simulink model "Motor_Position"  (R2020a)
settings: Solver=ode15s  StartTime=0.0  StopTime=0.2  RelTol=1e-3
undefined symbols (not defined in the file): b, J, K, Kd, Ki, Kp, L, R, Ts
settings Model: DataDictionary=Motordata.sldd  Creator=NIKITA  LastModifiedBy=NIKITA

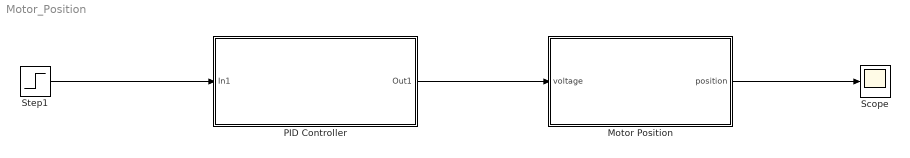
== system Motor_Position ==
  Motor Position : Subsystem
  PID Controller : Subsystem
  Scope : Scope
  Step1 : Step  Time=0  SampleTime=0
  wires:
  Motor Position/1(position) -> Scope/1
  Step1/1 -> PID Controller/1(In1)
  PID Controller/1(Out1) -> Motor Position/1(voltage)

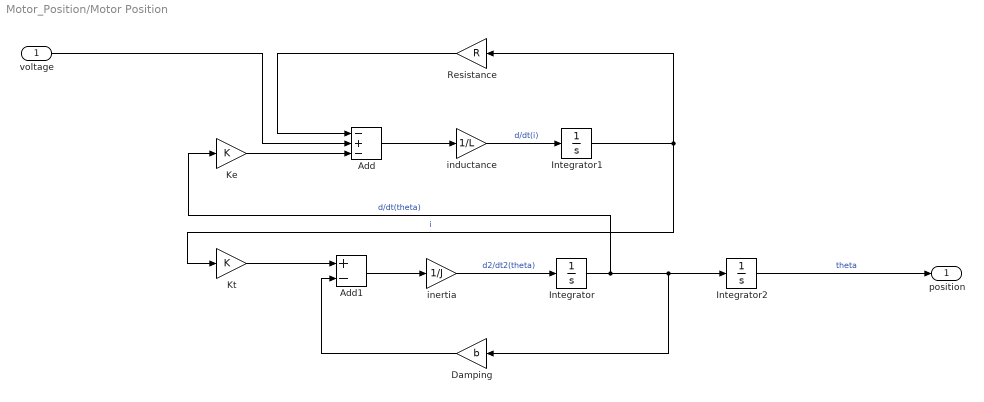
== system Motor_Position/Motor Position ==
  voltage : Inport
  Add : Sum  Inputs=-+-
  Add1 : Sum  Inputs=+-
  Damping : Gain  Gain=b
  "Integrator " : Integrator
  "Integrator1 " : Integrator
  "Integrator2 " : Integrator
  Ke : Gain  Gain=K
  Kt : Gain  Gain=K
  Resistance : Gain  Gain=R
  inductance : Gain  Gain=1/L
  inertia : Gain  Gain=1/J
  position : Outport
  wires:
  Add/1 -> inductance/1
  inertia/1 -> "Integrator "/1  "d2/dt2(theta)"
  Ke/1 -> Add/3
  Damping/1 -> Add1/2
  Resistance/1 -> Add/1
  "Integrator1 "/1 -> Resistance/1, Kt/1  "i"
  Kt/1 -> Add1/1
  "Integrator "/1 -> Ke/1, "Integrator2 "/1, Damping/1  "d/dt(theta)"
  voltage/1 -> Add/2
  inductance/1 -> "Integrator1 "/1  "d/dt(i)"
  Add1/1 -> inertia/1
  "Integrator2 "/1 -> position/1  "theta"

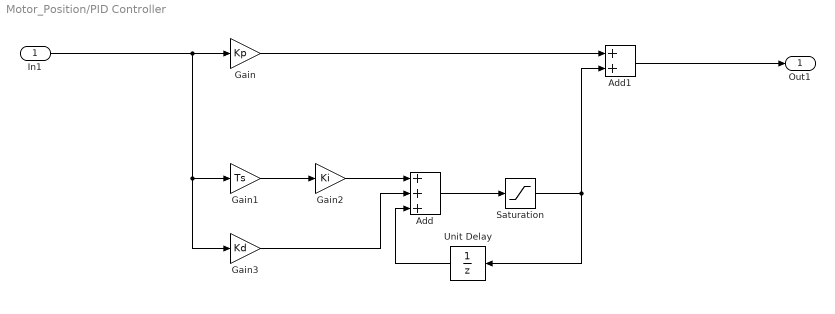
== system Motor_Position/PID Controller ==
  In1 : Inport
  Add : Sum  Inputs=+++
  Add1 : Sum
  Gain : Gain  Gain=Kp
  Gain1 : Gain  Gain=Ts
  Gain2 : Gain  Gain=Ki
  Gain3 : Gain  Gain=Kd
  Saturation : Saturate  UpperLimit=1  LowerLimit=-1
  Unit Delay : UnitDelay  SampleTime=-1  HasFrameUpgradeWarning=on
  Out1 : Outport
  wires:
  Unit Delay/1 -> Add/3
  Gain2/1 -> Add/1
  In1/1 -> Gain3/1, Gain1/1, Gain/1
  Gain/1 -> Add1/1
  Saturation/1 -> Add1/2, Unit Delay/1
  Gain1/1 -> Gain2/1
  Add1/1 -> Out1/1
  Add/1 -> Saturation/1
  Gain3/1 -> Add/2
